simulink model "pid_1dof_nonlinear_speed"  (R2017a)
settings: Solver=ode45  StartTime=0.0  StopTime=10  RelTol=1e-3
undefined symbols (not defined in the file): f, g, GoalPos, J, k_p, L, l, m_p
libraries: simulink x1
settings Model: Creator=sansh  LastModifiedBy=rj2318

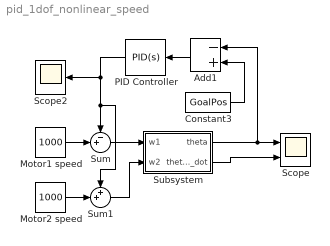
== system pid_1dof_nonlinear_speed ==
  Add1 : Sum  Inputs=-+
  Constant3 : Constant  Value=GoalPos
  Motor1 speed : Constant  Value=1000
  Motor2 speed : Constant  Value=1000
  PID Controller : simulink/Continuous/PID Controller  Controller=PID  TimeDomain=Continuous-time  SampleTime=-1  IntegratorMethod=Forward Euler  FilterMethod=Forward Euler  Form=Parallel  UseFilter=on  ControllerParametersSource=internal  P=50  I=0.01  D=1000  N=10  InitialConditionSource=internal  InitialConditionForIntegrator=0  InitialConditionForFilter=0  ExternalReset=none  LimitOutput=off  UpperSaturationLimit=inf  LowerSaturationLimit=-inf  LinearizeAsGain=on  AntiWindupMode=none  Kb=1  TrackingMode=off  Kt=1  PParamMin=[]  PParamMax=[]  IParamMin=[]  IParamMax=[]  DParamMin=[]  DParamMax=[]  NParamMin=[]  NParamMax=[]  KbParamMin=[]  KbParamMax=[]  KtParamMin=[]  KtParamMax=[]  POutMin=[]  POutMax=[]  IOutMin=[]  IOutMax=[]  DOutMin=[]  DOutMax=[]  NOutMin=[]  NOutMax=[]  KbOutMin=[]  KbOutMax=[]  KtOutMin=[]  KtOutMax=[]  IntegratorOutMin=[]  IntegratorOutMax=[]  FilterOutMin=[]  FilterOutMax=[]  SumOutMin=[]  SumOutMax=[]  SumI1OutMin=[]  SumI1OutMax=[]  SumI2OutMin=[]  SumI2OutMax=[]  SumI3OutMin=[]  SumI3OutMax=[]  SumDOutMin=[]  SumDOutMax=[]  SaturationOutMin=[]  SaturationOutMax=[]  IntegratorContinuousStateAttributes=''  IntegratorStateMustResolveToSignalObject=off  IntegratorRTWStateStorageClass=Auto  FilterContinuousStateAttributes=''  FilterStateMustResolveToSignalObject=off  FilterRTWStateStorageClass=Auto  DifferentiatorICPrevScaledInput=0  DifferentiatorOutMin=[]  DifferentiatorOutMax=[]  InitialConditionSetting=State (most efficient)
  Scope : Scope  NumInputPorts=2
  Scope2 : Scope
  Subsystem : Subsystem
  Sum : Sum  Inputs=-+|
  Sum1 : Sum  Inputs=++|
  wires:
  PID Controller/1 -> Sum1/1, Sum/1, Scope2/1
  Add1/1 -> PID Controller/1
  Subsystem/2(theta_dot) -> Scope/2
  Constant3/1 -> Add1/2
  Subsystem/1(theta) -> Scope/1, Add1/1
  Motor1 speed/1 -> Sum/2
  Motor2 speed/1 -> Sum1/2
  Sum/1 -> Subsystem/1(w1)
  Sum1/1 -> Subsystem/2(w2)

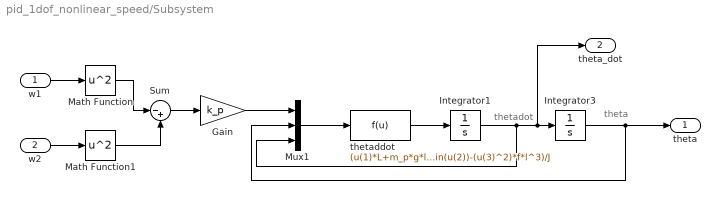
== system pid_1dof_nonlinear_speed/Subsystem ==
  note: theta
  note: thetadot
  w1 : Inport
  w2 : Inport  Port=2
  Gain : Gain  Gain=k_p
  Integrator1 : Integrator  ContinuousStateAttributes='thetadot'
  Integrator3 : Integrator  InitialCondition=pi  ContinuousStateAttributes='theta'
  Math Function : Math  Operator=square  SaturateOnIntegerOverflow=on
  Math Function1 : Math  Operator=square  SaturateOnIntegerOverflow=on
  Mux1 : Mux  Inputs=3
  Sum : Sum  Inputs=|-+
  thetaddot : Fcn  Expr=(u(1)*L+m_p*g*l*sin(u(2))-(u(3)^2)*f*l^3)/J
  theta : Outport
  theta_dot : Outport  Port=2
  wires:
  Mux1/1 -> thetaddot/1
  thetaddot/1 -> Integrator1/1
  Integrator1/1 -> Mux1/3, theta_dot/1, Integrator3/1
  Integrator3/1 -> Mux1/2, theta/1
  Gain/1 -> Mux1/1
  Sum/1 -> Gain/1
  w1/1 -> Math Function/1
  w2/1 -> Math Function1/1
  Math Function/1 -> Sum/1
  Math Function1/1 -> Sum/2
